simulink model "PhaseLockedLoop"  (R2014b)
settings: Solver=ode3  StartTime=0.0  StopTime=40  FixedStep=1e-2  MaxStep=1e-3  RelTol=1e-2
InitFcn:
  | PhaseLockedLoop_Initialization
values from neighbouring files (symbols this model uses):
  f = 2.9    [PhaseLockedLoop_Initialization.m]
  f_VCO = 4    [PhaseLockedLoop_Initialization.m]
undefined symbols (not defined in the file or in its folder): a, b
libraries: simulink x1, commsynccomp2 x1
settings Model: Creator=Vincent  LastModifiedBy=Vincent

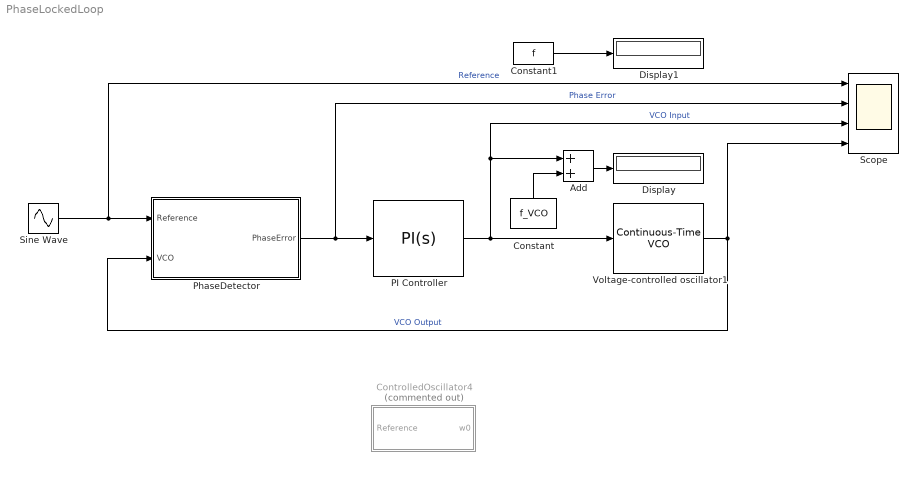
== system PhaseLockedLoop ==
  Add : Sum
  Constant : Constant  Value=f_VCO
  Constant1 : Constant  Value=f
  ControlledOscillator4 : Subsystem  Commented=on
  Display : Display
  Display1 : Display
  PI Controller : simulink/Continuous/PID Controller  Controller=PI  TimeDomain=Continuous-time  SampleTime=-1  IntegratorMethod=Forward Euler  FilterMethod=Forward Euler  Form=Parallel  P=1.5  I=0.8  D=0.1  N=100  InitialConditionSource=internal  InitialConditionForIntegrator=0  InitialConditionForFilter=0  ExternalReset=none  LimitOutput=off  UpperSaturationLimit=inf  LowerSaturationLimit=-inf  LinearizeAsGain=on  AntiWindupMode=none  Kb=1  TrackingMode=off  Kt=1  PParamMin=[]  PParamMax=[]  IParamMin=[]  IParamMax=[]  DParamMin=[]  DParamMax=[]  NParamMin=[]  NParamMax=[]  KbParamMin=[]  KbParamMax=[]  KtParamMin=[]  KtParamMax=[]  POutMin=[]  POutMax=[]  IOutMin=[]  IOutMax=[]  DOutMin=[]  DOutMax=[]  NOutMin=[]  NOutMax=[]  KbOutMin=[]  KbOutMax=[]  KtOutMin=[]  KtOutMax=[]  IntegratorOutMin=[]  IntegratorOutMax=[]  FilterOutMin=[]  FilterOutMax=[]  SumOutMin=[]  SumOutMax=[]  SumI1OutMin=[]  SumI1OutMax=[]  SumI2OutMin=[]  SumI2OutMax=[]  SumI3OutMin=[]  SumI3OutMax=[]  SumDOutMin=[]  SumDOutMax=[]  SaturationOutMin=[]  SaturationOutMax=[]  IntegratorContinuousStateAttributes=''  IntegratorStateMustResolveToSignalObject=off  IntegratorRTWStateStorageClass=Auto  FilterContinuousStateAttributes=''  FilterStateMustResolveToSignalObject=off  FilterRTWStateStorageClass=Auto  DifferentiatorICPrevScaledInput=0  DifferentiatorOutMin=[]  DifferentiatorOutMax=[]  UseFilter=on
  PhaseDetector : Subsystem
  Scope : Scope  NumInputPorts=4
      settings: TimeRange=8  YMin=-5~0.660714~-5~-5  YMax=5~4.66071~5~5
  Sine Wave : Sin  Frequency=f*2*pi  SampleTime=0
  Voltage-controlled oscillator1 : commsynccomp2/Continuous-Time VCO  Ac=1  Fc=f_VCO  Kc=1  Ph=0
  wires:
  Voltage-controlled oscillator1/1 -> Scope/4, PhaseDetector/2(VCO)  "VCO Output"
  Sine Wave/1 -> Scope/1, PhaseDetector/1(Reference)  "Reference"
  PI Controller/1 -> Voltage-controlled oscillator1/1, Scope/3, Add/1  "VCO Input"
  PhaseDetector/1(PhaseError) -> PI Controller/1, Scope/2  "Phase Error"
  Add/1 -> Display/1
  Constant/1 -> Add/2
  Constant1/1 -> Display1/1

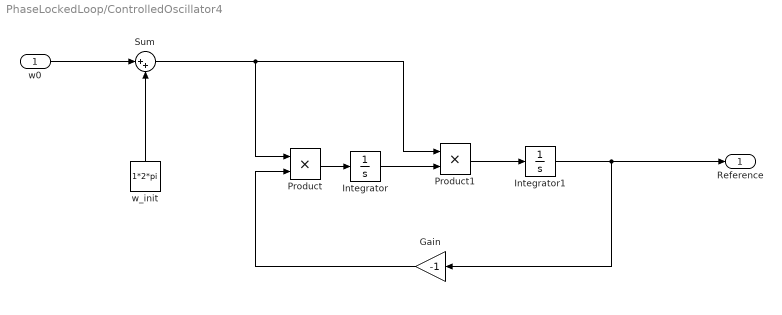
== system PhaseLockedLoop/ControlledOscillator4 ==
  w0 : Inport
  Gain : Gain  Gain=-1
  Integrator : Integrator
  Integrator1 : Integrator
  Product : Product
  Product1 : Product
  Sum : Sum  Inputs=|++
  w_init : Constant  Value=1*2*pi
  Reference : Outport
  wires:
  w0/1 -> Sum/1
  w_init/1 -> Sum/2
  Sum/1 -> Product/1, Product1/1
  Product/1 -> Integrator/1
  Integrator/1 -> Product1/2
  Product1/1 -> Integrator1/1
  Integrator1/1 -> Reference/1, Gain/1
  Gain/1 -> Product/2

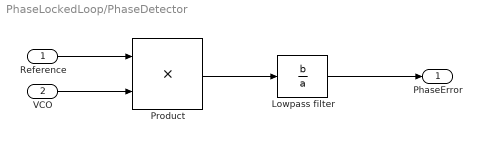
== system PhaseLockedLoop/PhaseDetector ==
  Reference : Inport
  VCO : Inport  Port=2
  Lowpass filter : TransferFcn  Numerator=b  Denominator=a
  Product : Product
  PhaseError : Outport
  wires:
  VCO/1 -> Product/2
  Reference/1 -> Product/1
  Lowpass filter/1 -> PhaseError/1
  Product/1 -> Lowpass filter/1
